simulink model "mancal_v2_corsi_simu"  (R2013a)
settings: Solver=ode45  StartTime=0.0  StopTime=0.7  RelTol=1e-5
values from neighbouring files (symbols this model uses):
  c = tf(Num,Den)    [parametrizaControlador.m]
  dA = [1.435e2 3.335e-2]    [parametriza.m]    (also in parametrizaMancal.m)
  E = 3e9    (= 3000000000)    [parametriza.m]    (also in parametrizaMancal.m)
  gb = 0.3e-3    (= 0.0003)    [parametriza.m]    (also in parametrizaMancal.m)
  gi = 0.7e-3    (= 0.0007)    [parametriza.m]    (also in parametrizaMancal.m)
  Hb = 8e-3    (= 0.008)    [parametriza.m]    (also in parametrizaMancal.m)
  Kb = 58    [parametriza.m]    (also in parametrizaMancal.m = E*Hb*Ab/Lb)
  Ke = [3.8e-9 2.86e-3]    [parametrizaMancal.m]
  Km = 600e3    (= 600000)    [parametrizaMancal.m]
  L = tf(Kb,[L2 R])    [parametriza.m]    (also in parametrizaMancal.m = [0 L(1)*gi + L(2)])
  Lb = 5.3e-3    (= 0.0053)    [parametriza.m]    (also in parametrizaMancal.m)
  m = 0.375    [parametriza.m]    (also in parametrizaMancal.m)
  N = 300    [parametriza.m]    (also in parametrizaMancal.m)
  R = 6.3    [parametriza.m]    (also in parametrizaMancal.m = 6)
  Vmax = 30    [parametriza.m]    (also in parametrizaMancal.m)
libraries: simulink x1, dspmathops x1
settings Model: Creator=leo  LastModifiedBy=rafa
settings OptimizationCC: AccelVerboseBuild=on
settings DebuggingCC: SolverPrmCheckMsg=none
settings ModelReferenceCC: UpdateModelReferenceTargets=IfOutOfDate
settings SFSimCC: SFSimEcho=off

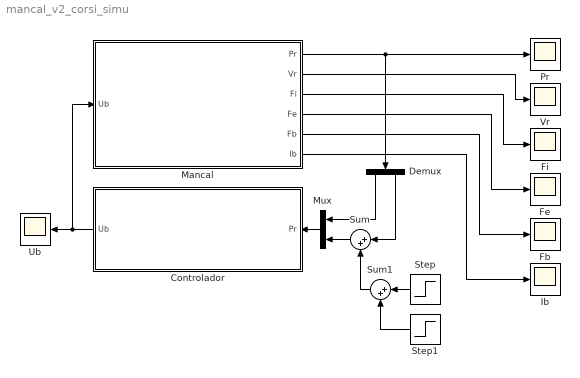
== system mancal_v2_corsi_simu ==
  Controlador : Subsystem
  Demux : Demux  Outputs=2
  Fb : Scope
      settings: YMin=-200000  YMax=200000  SaveName=ScopeData6
  Fe : Scope
      settings: YMin=-500  YMax=25  SaveName=ScopeData2
  Fi : Scope
      settings: YMin=0  YMax=450  SaveName=ScopeData3
  Ib : Scope
      settings: YMin=-4  YMax=4  SaveName=ScopeData5
  Mancal : Subsystem
  Mux : Mux  Inputs=2
  Pr : Scope
      settings: TimeRange=1  YMin=-7.5e-05  YMax=0.000375  SaveName=pr
  Step : Step  Time=0.5  After=5E-6  SampleTime=0
  Step1 : Step  Time=0.55  After=-5E-6  SampleTime=0
  Sum : Sum  Inputs=|++
  Sum1 : Sum  Inputs=|++
  Ub : Scope
      settings: TimeRange=0.1  YMin=0  YMax=10  SaveName=ScopeData10
  Vr : Scope
      settings: YMin=-45  YMax=45
  wires:
  Mancal/1(Pr) -> Demux/1, Pr/1
  Mancal/2(Vr) -> Vr/1
  Mancal/4(Fe) -> Fe/1
  Mancal/3(Fi) -> Fi/1
  Mancal/6(Ib) -> Ib/1
  Mancal/5(Fb) -> Fb/1
  Controlador/1(Ub) -> Ub/1, Mancal/1(Ub)
  Step/1 -> Sum1/1
  Sum1/1 -> Sum/2
  Step1/1 -> Sum1/2
  Mux/1 -> Controlador/1(Pr)
  Demux/1 -> Mux/1
  Sum/1 -> Mux/2
  Demux/2 -> Sum/1

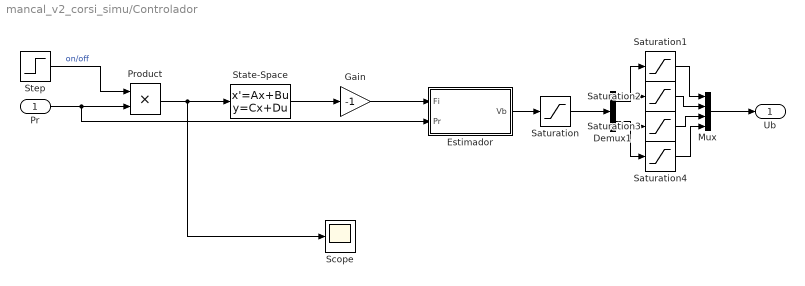
== system mancal_v2_corsi_simu/Controlador ==
  Pr : Inport
  Demux1 : Demux  Outputs=2
  Estimador : Subsystem
  Gain : Gain  Gain=-1
  Mux : Mux
  Product : Product
  Saturation : Saturate  UpperLimit=Vmax  LowerLimit=-Vmax
  Saturation1 : Saturate  UpperLimit=Inf  LowerLimit=0
  Saturation2 : Saturate  UpperLimit=0  LowerLimit=-Inf
  Saturation3 : Saturate  UpperLimit=Inf  LowerLimit=0
  Saturation4 : Saturate  UpperLimit=0  LowerLimit=-Inf
  Scope : Scope
      settings: YMin=-2.5e-05  YMax=2e-05  SaveName=ScopeData20
  State-Space : StateSpace  A=ss([c 1; 1 c]).A  B=ss([c 1; 1 c]).B  C=ss([c 1; 1 c]).C  D=ss([c 1; 1 c]).D
  Step : Step  Time=0.1  SampleTime=0
  Ub : Outport
  wires:
  Mux/1 -> Ub/1
  Saturation/1 -> Demux1/1
  Saturation4/1 -> Mux/4
  Saturation3/1 -> Mux/3
  Saturation2/1 -> Mux/2
  Saturation1/1 -> Mux/1
  Demux1/2 -> Saturation3/1, Saturation4/1
  Demux1/1 -> Saturation2/1, Saturation1/1
  Gain/1 -> Estimador/1(Fi)
  Estimador/1(Vb) -> Saturation/1
  State-Space/1 -> Gain/1
  Product/1 -> Scope/1, State-Space/1
  Pr/1 -> Product/2, Estimador/2(Pr)
  Step/1 -> Product/1  "on/off"

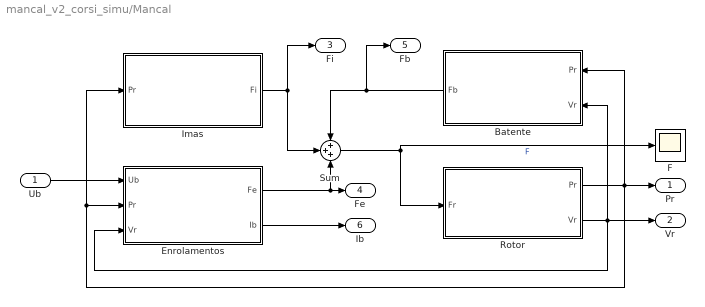
== system mancal_v2_corsi_simu/Mancal ==
  Ub : Inport
  Batente : Subsystem
  Enrolamentos : Subsystem
  F : Scope
      settings: TimeRange=1  YMin=-200000  YMax=200000  SaveName=ScopeData13
  Imas : Subsystem
  Rotor : Subsystem
  Sum : Sum  Inputs=+++
  Pr : Outport
  Vr : Outport  Port=2
  Fi : Outport  Port=3
  Fe : Outport  Port=4
  Fb : Outport  Port=5
  Ib : Outport  Port=6
  wires:
  Sum/1 -> Rotor/1(Fr), F/1  "F"
  Ub/1 -> Enrolamentos/1(Ub)
  Enrolamentos/1(Fe) -> Sum/3, Fe/1
  Enrolamentos/2(Ib) -> Ib/1
  Batente/1(Fb) -> Sum/1, Fb/1
  Rotor/1(Pr) -> Batente/1(Pr), Pr/1, Enrolamentos/2(Pr), Imas/1(Pr)
  Rotor/2(Vr) -> Enrolamentos/3(Vr), Batente/2(Vr), Vr/1
  Imas/1(Fi) -> Sum/2, Fi/1

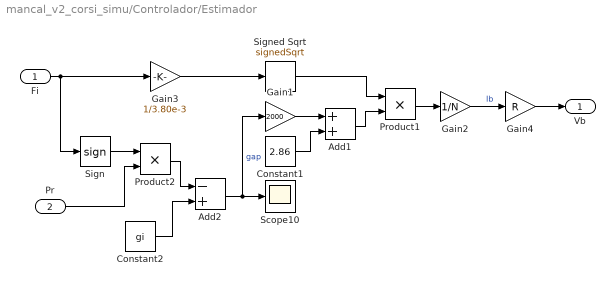
== system mancal_v2_corsi_simu/Controlador/Estimador ==
  Fi : Inport
  Pr : Inport  Port=2
  Add1 : Sum
  Add2 : Sum  Inputs=-+
  Constant1 : Constant  Value=2.86
  Constant2 : Constant  Value=gi
  Gain1 : Gain  Gain=2000
  Gain2 : Gain  Gain=1/N
  Gain3 : Gain  Gain=1/3.80e-3
  Gain4 : Gain  Gain=R
  Product1 : Product
  Product2 : Product
  Scope10 : Scope
      settings: TimeRange=2.85171102661597  YMin=0.00015  YMax=0.0006  SaveName=ScopeData11
  Sign : Signum
  Signed Sqrt : Sqrt  Operator=signedSqrt  SaturateOnIntegerOverflow=on
  Vb : Outport
  wires:
  Constant2/1 -> Add2/2
  Product2/1 -> Add2/1
  Pr/1 -> Product2/2
  Sign/1 -> Product2/1
  Gain4/1 -> Vb/1
  Product1/1 -> Gain2/1
  Add2/1 -> Scope10/1, Gain1/1  "gap"
  Constant1/1 -> Add1/2
  Signed Sqrt/1 -> Product1/1
  Gain2/1 -> Gain4/1  "Ib"
  Gain3/1 -> Signed Sqrt/1
  Gain1/1 -> Add1/1
  Fi/1 -> Sign/1, Gain3/1
  Add1/1 -> Product1/2

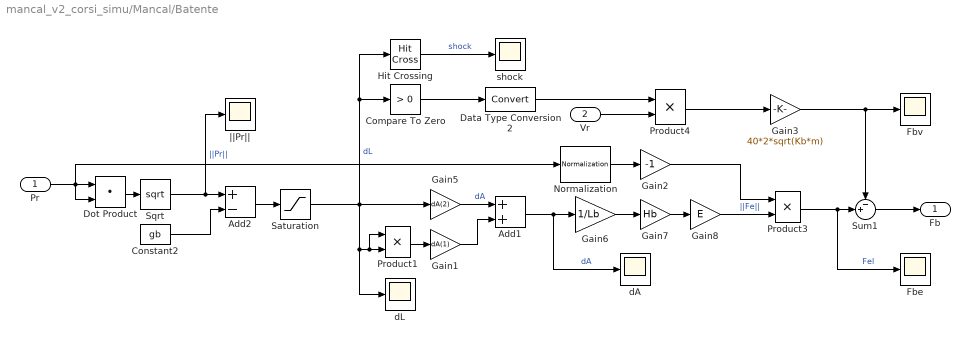
== system mancal_v2_corsi_simu/Mancal/Batente ==
  Pr : Inport
  Vr : Inport  Port=2
  Add1 : Sum
  Add2 : Sum  Inputs=+-
  Compare To Zero : simulink/Logic and Bit Operations/Compare To Zero  relop=>  OutDataTypeStr=boolean
  Constant2 : Constant  Value=gb
  Data Type Conversion2 : DataTypeConversion
  Dot Product : DotProduct  InputSameDT=on  OutDataTypeStr=Inherit: Inherit via internal rule
  Fbe : Scope
      settings: TimeRange=0.0002829354553492485  YMin=-100000  YMax=100000  SaveName=ScopeData15
  Fbv : Scope
      settings: TimeRange=0.1  YMin=-225000  YMax=225000  SaveName=ScopeData8
  Gain1 : Gain  Gain=dA(1)
  Gain2 : Gain  Gain=-1
  Gain3 : Gain  Gain=40*2*sqrt(Kb*m)
  Gain5 : Gain  Gain=dA(2)
  Gain6 : Gain  Gain=1/Lb
  Gain7 : Gain  Gain=Hb
  Gain8 : Gain  Gain=E
  Hit Crossing : HitCross  HitCrossingDirection=rising
  Normalization : dspmathops/Normalization  NormType=2-norm  Bias=1e-10  NormOver=Each column  ColComp=on  Dimension=1  outputDataTypeStr=Inherit: Same as product output  outputLastDataTypeStr=Inherit: Same as product output  outputMin=[]  outputMax=[]  accumDataTypeStr=Inherit: Same as product output  accumLastDataTypeStr=Inherit: Same as product output  roundingMode=Floor  overflowMode=off
  Product1 : Product
  Product3 : Product
  Product4 : Product
  Saturation : Saturate  UpperLimit=Inf  LowerLimit=0
  Sqrt : Sqrt  SaturateOnIntegerOverflow=on
  Sum1 : Sum  Inputs=-+|
  dA : Scope
      settings: TimeRange=0.0002829354553492485  YMin=3.91545e-05  YMax=3.9158e-05  SaveName=ScopeData4
  dL : Scope
      settings: TimeRange=0.1  YMin=1.4215e-06  YMax=1.4315e-06  SaveName=ScopeData7
  shock : Scope
      settings: TimeRange=0.0002829354553492485  YMin=5.54637e-16  YMax=5.54639e-16  SaveName=ScopeData19
  ||Pr|| : Scope
      settings: TimeRange=0.0002829354553492485  YMin=-2.75  YMax=0  SaveName=ScopeData18
  Fb : Outport
  wires:
  Dot Product/1 -> Sqrt/1
  Gain8/1 -> Product3/2  "||Fe||"
  Compare To Zero/1 -> Data Type Conversion2/1
  Saturation/1 -> dL/1, Product1/1, Product1/2, Hit Crossing/1, Compare To Zero/1, Gain5/1  "dL"
  Add2/1 -> Saturation/1
  Sqrt/1 -> ||Pr||/1, Add2/1  "||Pr||"
  Constant2/1 -> Add2/2
  Gain6/1 -> Gain7/1
  Gain7/1 -> Gain8/1
  Product4/1 -> Gain3/1
  Product3/1 -> Sum1/2, Fbe/1  "Fel"
  Sum1/1 -> Fb/1
  Data Type Conversion2/1 -> Product4/1
  Product1/1 -> Gain1/1
  Gain5/1 -> Add1/1  "dA"
  Add1/1 -> dA/1, Gain6/1  "dA"
  Gain3/1 -> Fbv/1, Sum1/1
  Vr/1 -> Product4/2
  Normalization/1 -> Gain2/1
  Pr/1 -> Normalization/1, Dot Product/2, Dot Product/1
  Gain2/1 -> Product3/1
  Gain1/1 -> Add1/2
  Hit Crossing/1 -> shock/1  "shock"

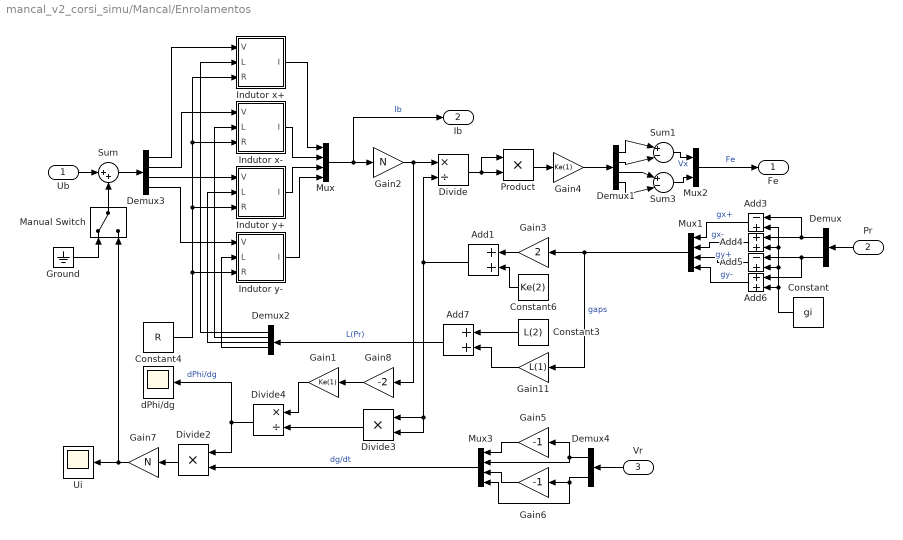
== system mancal_v2_corsi_simu/Mancal/Enrolamentos ==
  Ub : Inport
  Pr : Inport  Port=2
  Vr : Inport  Port=3
  Add{1,4,6..7} (4 alike) : Sum
  Add3 : Sum  Inputs=-+
  Add5 : Sum  Inputs=-+
  Constant : Constant  Value=gi
  Constant3 : Constant  Value=L(2)
  Constant4 : Constant  Value=R
  Constant6 : Constant  Value=Ke(2)
  Demux : Demux  Outputs=2
  Demux1 : Demux
  Demux2 : Demux
  Demux3 : Demux
  Demux4 : Demux  Outputs=2
  Divide : Product  Inputs=*/
  Divide2 : Product  Inputs=**
  Divide3 : Product  Inputs=**
  Divide4 : Product  Inputs=*/
  Gain1 : Gain  Gain=Ke(1)
  Gain11 : Gain  Gain=L(1)
  Gain2 : Gain  Gain=N
  Gain3 : Gain  Gain=2
  Gain4 : Gain  Gain=Ke(1)
  Gain5 : Gain  Gain=-1
  Gain6 : Gain  Gain=-1
  Gain7 : Gain  Gain=N
  Gain8 : Gain  Gain=-2
  Ground : Ground
  Indutor x+ : Subsystem
  Indutor x- : Subsystem
  Indutor y+ : Subsystem
  Indutor y- : Subsystem
  Manual Switch : ManualSwitch
  Mux : Mux
  Mux1 : Mux
  Mux2 : Mux  Inputs=2
  Mux3 : Mux
  Product : Product
  Sum : Sum  Inputs=|++
  Sum1 : Sum  Inputs=|+-|
  Sum3 : Sum  Inputs=|+-|
  Ui : Scope
      settings: TimeRange=0.0002829354553492485  YMin=-175  YMax=175  SaveName=ScopeData12
  dPhi/dg : Scope
      settings: TimeRange=0.0002829354553492485  YMin=-100000  YMax=100000  SaveName=ScopeData14
  Fe : Outport
  Ib : Outport  Port=2
  wires:
  Add1/1 -> Divide3/2, Divide3/1, Divide/2
  Gain2/1 -> Gain8/1, Divide/1
  Product/1 -> Gain4/1
  Gain3/1 -> Add1/1
  Constant/1 -> Add5/2, Add4/2, Add3/2, Add6/2
  Constant6/1 -> Add1/2
  Divide/1 -> Product/2, Product/1
  Mux/1 -> Ib/1, Gain2/1  "Ib"
  Demux1/2 -> Sum1/2
  Demux3/3 -> Indutor y+/1(V)
  Demux3/2 -> Indutor x-/1(V)
  Indutor x-/1(I) -> Mux/2
  Indutor y+/1(I) -> Mux/3
  Indutor y-/1(I) -> Mux/4
  Gain4/1 -> Demux1/1
  Mux2/1 -> Fe/1  "Fe"
  Sum3/1 -> Mux2/2
  Sum1/1 -> Mux2/1  "Vx"
  Demux1/4 -> Sum3/2
  Demux1/1 -> Sum1/1
  Demux1/3 -> Sum3/1
  Add3/1 -> Mux1/1  "gx+"
  Add4/1 -> Mux1/2  "gx-"
  Add5/1 -> Mux1/3  "gy+"
  Add6/1 -> Mux1/4  "gy-"
  Mux1/1 -> Gain3/1, Gain11/1  "gaps"
  Demux/1 -> Add4/1, Add3/1
  Demux/2 -> Add5/1, Add6/1
  Demux3/4 -> Indutor y-/1(V)
  Add7/1 -> Demux2/1  "L(Pr)"
  Constant4/1 -> Indutor x+/3(R), Indutor x-/3(R), Indutor y+/3(R), Indutor y-/3(R)
  Constant3/1 -> Add7/1
  Gain11/1 -> Add7/2
  Demux2/2 -> Indutor x-/2(L)
  Demux2/3 -> Indutor y+/2(L)
  Demux2/4 -> Indutor y-/2(L)
  Indutor x+/1(I) -> Mux/1
  Demux2/1 -> Indutor x+/2(L)
  Pr/1 -> Demux/1
  Demux3/1 -> Indutor x+/1(V)
  Divide2/1 -> Gain7/1
  Vr/1 -> Demux4/1
  Demux4/1 -> Mux3/2, Gain5/1
  Gain5/1 -> Mux3/1
  Gain6/1 -> Mux3/3
  Mux3/1 -> Divide2/2  "dg/dt"
  Gain7/1 -> Manual Switch/2, Ui/1
  Gain8/1 -> Gain1/1
  Gain1/1 -> Divide4/1
  Divide3/1 -> Divide4/2
  Divide4/1 -> Divide2/1, dPhi/dg/1  "dPhi/dg"
  Demux4/2 -> Mux3/4, Gain6/1
  Ub/1 -> Sum/1
  Sum/1 -> Demux3/1
  Manual Switch/1 -> Sum/2
  Ground/1 -> Manual Switch/1

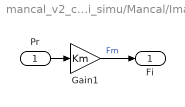
== system mancal_v2_corsi_simu/Mancal/Imas ==
  Pr : Inport
  Gain1 : Gain  Gain=Km
  Fi : Outport
  wires:
  Pr/1 -> Gain1/1
  Gain1/1 -> Fi/1  "Fm"

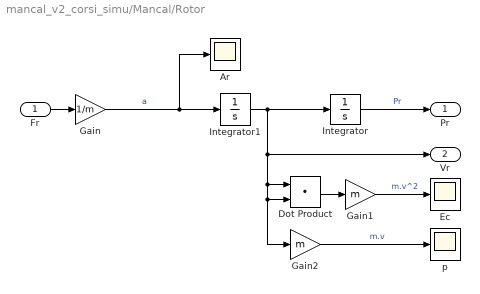
== system mancal_v2_corsi_simu/Mancal/Rotor ==
  Fr : Inport
  Ar : Scope
      settings: TimeRange=1  YMin=-200000  YMax=200000  SaveName=ScopeData9
  Dot Product : DotProduct  InputSameDT=on  OutDataTypeStr=Inherit: Inherit via internal rule
  Ec : Scope
      settings: TimeRange=0.25  YMin=0  YMax=0.09  SaveName=ScopeData16
  Gain : Gain  Gain=1/m
  Gain1 : Gain  Gain=m
  Gain2 : Gain  Gain=m
  Integrator : Integrator  InitialCondition=[.001 .002]*1e-3  UpperSaturationLimit=Inf  LowerSaturationLimit=-Inf
  Integrator1 : Integrator
  p : Scope
      settings: TimeRange=1  YMin=-200000  YMax=200000  SaveName=ScopeData17
  Pr : Outport
  Vr : Outport  Port=2
  wires:
  Fr/1 -> Gain/1
  Integrator/1 -> Pr/1  "Pr"
  Gain/1 -> Ar/1, Integrator1/1  "a"
  Dot Product/1 -> Gain1/1
  Integrator1/1 -> Dot Product/1, Gain2/1, Dot Product/2, Vr/1, Integrator/1
  Gain2/1 -> p/1  "m.v"
  Gain1/1 -> Ec/1  "m.v^2"

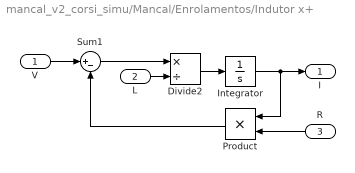
== system mancal_v2_corsi_simu/Mancal/Enrolamentos/Indutor x+ ==
  V : Inport
  L : Inport  Port=2
  R : Inport  Port=3
  Divide2 : Product  Inputs=*/
  Integrator : Integrator
  Product : Product
  Sum1 : Sum  Inputs=|+-
  I : Outport
  wires:
  Divide2/1 -> Integrator/1
  Sum1/1 -> Divide2/1
  Integrator/1 -> Product/1, I/1
  Product/1 -> Sum1/2
  L/1 -> Divide2/2
  V/1 -> Sum1/1
  R/1 -> Product/2

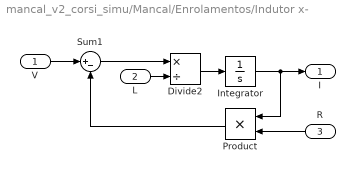
== system mancal_v2_corsi_simu/Mancal/Enrolamentos/Indutor x- ==
  V : Inport
  L : Inport  Port=2
  R : Inport  Port=3
  Divide2 : Product  Inputs=*/
  Integrator : Integrator
  Product : Product
  Sum1 : Sum  Inputs=|+-
  I : Outport
  wires:
  R/1 -> Product/2
  V/1 -> Sum1/1
  L/1 -> Divide2/2
  Product/1 -> Sum1/2
  Integrator/1 -> I/1, Product/1
  Sum1/1 -> Divide2/1
  Divide2/1 -> Integrator/1

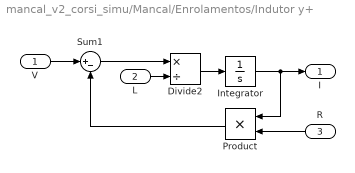
== system mancal_v2_corsi_simu/Mancal/Enrolamentos/Indutor y+ ==
  V : Inport
  L : Inport  Port=2
  R : Inport  Port=3
  Divide2 : Product  Inputs=*/
  Integrator : Integrator
  Product : Product
  Sum1 : Sum  Inputs=|+-
  I : Outport
  wires:
  R/1 -> Product/2
  V/1 -> Sum1/1
  L/1 -> Divide2/2
  Product/1 -> Sum1/2
  Integrator/1 -> I/1, Product/1
  Sum1/1 -> Divide2/1
  Divide2/1 -> Integrator/1

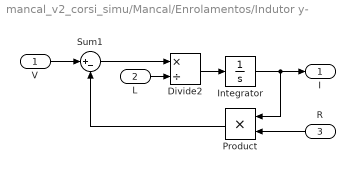
== system mancal_v2_corsi_simu/Mancal/Enrolamentos/Indutor y- ==
  V : Inport
  L : Inport  Port=2
  R : Inport  Port=3
  Divide2 : Product  Inputs=*/
  Integrator : Integrator
  Product : Product
  Sum1 : Sum  Inputs=|+-
  I : Outport
  wires:
  R/1 -> Product/2
  V/1 -> Sum1/1
  L/1 -> Divide2/2
  Product/1 -> Sum1/2
  Integrator/1 -> I/1, Product/1
  Sum1/1 -> Divide2/1
  Divide2/1 -> Integrator/1
